simulink model "Hybrid_VTOL"  (R2024a)
settings: Solver=ode4  StartTime=0.0  StopTime=inf  FixedStep=1/100  RelTol=1e-3
libraries: shared6dof x1, sharedtransform x1, simulink_extras x1, dspnetwork x1
settings Model: Creator=cyber  LastModifiedBy=cyber

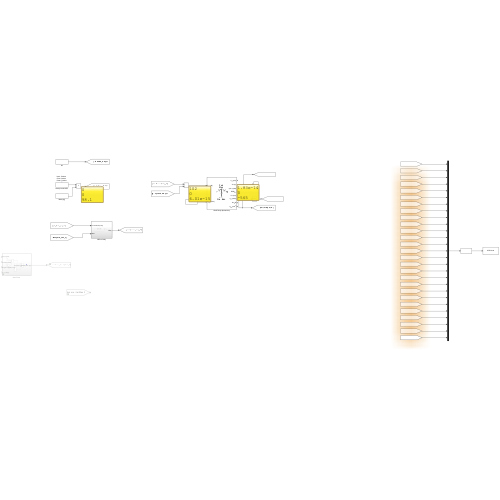
[thumbnail: Simulink's stored preview of the top-level diagram]
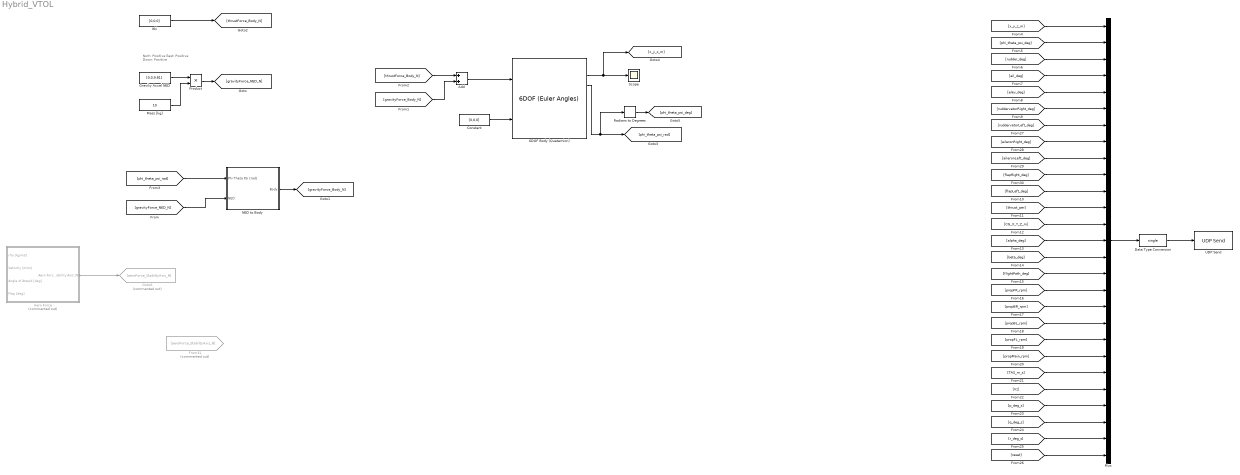
== system Hybrid_VTOL ==
  note: Norh: Positive
      | East: Positive
      | Down: Positive
  6DOF Body (Quaternion) : shared6dof/6DOF (Euler Angles)  units=Metric (MKS)  mtype=Fixed  rep=Quaternion  xme_0=[0 0 -500]  Vm_0=[0 0 0]  eul_0=deg2rad([0 0 0])  pm_0=[0 0 0]  mass_0=1.0  mass_e=0.5  mass_f=2.0  inertia=eye(3)  inertia_e=eye(3)  inertia_f=2*eye(3)  k_quat=1.0  vre_flag=on  abi_flag=off  aMode=0  xme_statename=''  Vm_statename=''  eul_statename=''  quat_statename=''  pm_statename=''  mass_statename=''
      settings: LibrarySourceBlock=aerolib6dof2/6DOF (Quaternion)
  Add : Sum
  "Aero Force " : Subsystem  Commented=on
  Constant : Constant  Value=[0,0,0]
  Data Type Conversion : DataTypeConversion  OutDataTypeStr=single  SaturateOnIntegerOverflow=off  RndMeth=Floor
  From31 : From  Commented=on  GotoTag=aeroForce_StabiltyAxis_N
  Goto6 : Goto  Commented=on  GotoTag=aeroForce_StabiltyAxis_N
  "Gravity Accel NED " : Constant  Value=[0,0,9.81]
  Itki : Constant  Value=[0,0,0]
  Mass [kg] : Constant  Value=10
  Mux : Mux  Inputs=27
  NED to Body : Subsystem
  Product : Product
  Radians to Degrees : simulink_extras/Transformations/Radians to Degrees
  Scope : Scope
  UDP Send : dspnetwork/UDP Send  remoteURL='127.0.0.5'  remotePort=8005  localURL='0.0.0.0'  localPortSource=Automatically determine  localPort=-1  sendBufferSize=50*4  sampletime=-1  blockPlatform=[]  separateLengthPort=0
  wires:
  "Gravity Accel NED "/1 -> Product/1
  Mass [kg]/1 -> Product/2
  Product/1 -> [gravityForce_NED_N]
  [phi_theta_psi_rad] -> NED to Body/1(Phi Theta Psi [rad])
  [gravityForce_NED_N] -> NED to Body/2(NED)
  NED to Body/1(Body) -> [gravityForce_Body_N]
  Itki/1 -> [thrustForce_Body_N]
  [thrustForce_Body_N] -> Add/1
  [gravityForce_Body_N] -> Add/2
  Add/1 -> 6DOF Body (Quaternion)/1
  6DOF Body (Quaternion)/3 -> Radians to Degrees/1, [phi_theta_psi_rad]
  6DOF Body (Quaternion)/2 -> [x_y_z_m], Scope/1
  [r_deg_s] -> Mux/26
  [alpha_deg] -> Mux/14
  [propFR_rpm] -> Mux/17
  [x_y_z_m] -> Mux/1
  [elev_deg] -> Mux/5
  [thrust_per] -> Mux/12
  [q_deg_s] -> Mux/25
  [ruddervatorRight_deg] -> Mux/6
  [Vz] -> Mux/23
  Data Type Conversion/1 -> UDP Send/1
  [aileronRight_deg] -> Mux/8
  [flapLeft_deg] -> Mux/11
  [ail_deg] -> Mux/4
  [propFL_rpm] -> Mux/20
  [phi_theta_psi_deg] -> Mux/2
  [ruddervatorLeft_deg] -> Mux/7
  Mux/1 -> Data Type Conversion/1
  [p_deg_s] -> Mux/24
  [reset] -> Mux/27
  [rudder_deg] -> Mux/3
  [aileronLeft_deg] -> Mux/9
  [propBR_rpm] -> Mux/18
  [beta_deg] -> Mux/15
  [propBL_rpm] -> Mux/19
  [propMain_rpm] -> Mux/21
  [flightPath_deg] -> Mux/16
  [CG_X_Y_Z_m] -> Mux/13
  [TAS_m_s] -> Mux/22
  [flapRight_deg] -> Mux/10
  Radians to Degrees/1 -> [phi_theta_psi_deg]
  Constant/1 -> 6DOF Body (Quaternion)/2
  "Aero Force "/1(Aero Force Stability Axis [N]) -> Goto6/1

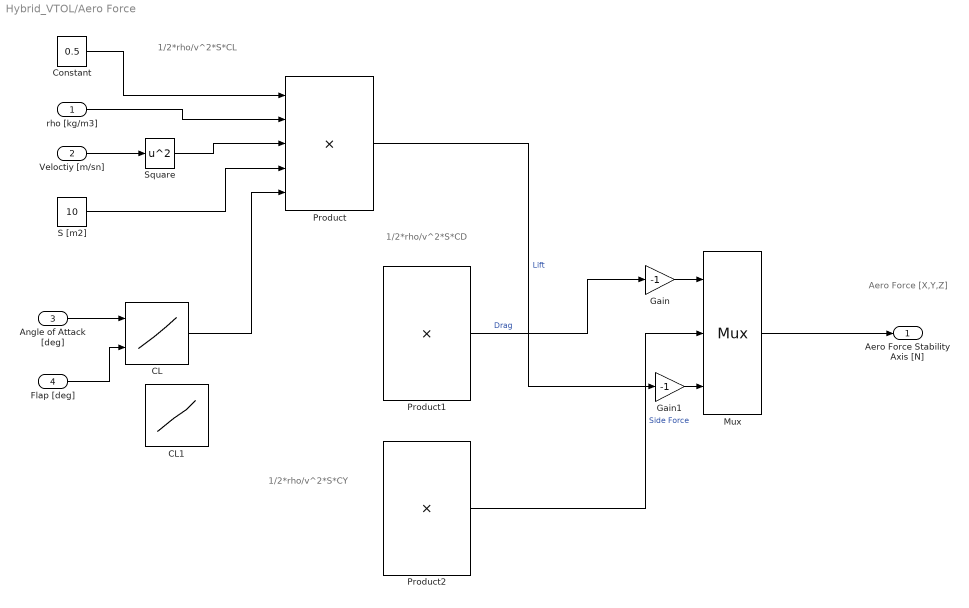
== system Hybrid_VTOL/Aero Force  ==
  note: Aero Force [X,Y,Z]
  note: 1/2*rho/v^2*S*CL
  note: 1/2*rho/v^2*S*CD
  note: 1/2*rho/v^2*S*CY
  rho [kg/m3] : Inport
  Veloctiy [m/sn] : Inport  Port=2
  Angle of Attack [deg] : Inport  Port=3
  Flap [deg] : Inport  Port=4
  CL : Lookup_n-D  BreakpointsForDimension1=[-5:5]  Table=tanh([-5:5])  InterpMethod=Linear Lagrange  InternalRulePriority=Speed  RndMeth=Simplest
      settings: InputPortMap=u0,u1
  CL1 : Lookup_n-D  BreakpointsForDimension1=[-5:5]  Table=tanh([-5:5])  InterpMethod=Linear Lagrange  InternalRulePriority=Speed  RndMeth=Simplest
      settings: InputPortMap=u0,u1
  Constant : Constant  Value=0.5
  Gain : Gain  Gain=-1
  Gain1 : Gain  Gain=-1
  Mux : Mux  Inputs=3
  Product : Product  Inputs=5
  Product1 : Product  Inputs=5
  Product2 : Product  Inputs=5
  S [m2] : Constant  Value=10
  Square : Math  Operator=square
  Aero Force Stability Axis [N] : Outport
  wires:
  Veloctiy [m/sn]/1 -> Square/1
  Angle of Attack [deg]/1 -> CL/1
  Flap [deg]/1 -> CL/2
  CL/1 -> Product/5
  S [m2]/1 -> Product/4
  Constant/1 -> Product/1
  rho [kg/m3]/1 -> Product/2
  Square/1 -> Product/3
  Product/1 -> Gain1/1  "Lift"
  Product1/1 -> Gain/1  "Drag"
  Gain/1 -> Mux/1
  Product2/1 -> Mux/2  "Side Force"
  Gain1/1 -> Mux/3
  Mux/1 -> Aero Force Stability Axis [N]/1

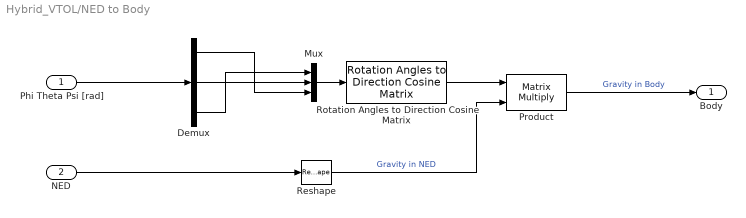
== system Hybrid_VTOL/NED to Body ==
  Phi Theta Psi [rad] : Inport
  NED : Inport  Port=2
  Demux : Demux  Outputs=3
  Mux : Mux  Inputs=3
  Product : Product  Multiplication=Matrix(*)
  Reshape : Reshape  OutputDimensionality=Column vector (2-D)
  Rotation Angles to Direction Cosine Matrix : sharedtransform/Rotation Angles to Direction Cosine Matrix  rotationOrder=ZYX  aMode=aMode
  Body : Outport
  wires:
  Mux/1 -> Rotation Angles to Direction Cosine Matrix/1
  Reshape/1 -> Product/2  "Gravity in NED"
  Demux/2 -> Mux/2
  Phi Theta Psi [rad]/1 -> Demux/1
  NED/1 -> Reshape/1
  Demux/1 -> Mux/3
  Demux/3 -> Mux/1
  Rotation Angles to Direction Cosine Matrix/1 -> Product/1
  Product/1 -> Body/1  "Gravity in Body"
